simulink model "GMCLIB_ClarkInv_BAM_F32"  (Simulink 7.3)
settings: Solver=ode45  StartTime=0.0  StopTime=10.0  RelTol=1e-3
settings Model: Creator=B17364  LastModifiedBy=B17364

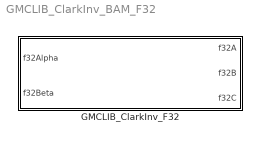
== system GMCLIB_ClarkInv_BAM_F32 ==
  GMCLIB_ClarkInv_F32 : Subsystem  mask(GMCLIB_ClarkInv_F32){}
      mask help: Bit accurate model of inverse Clarke transformation 2ph -> 3ph
      mask init:
      | pos = get_param(gcb, 'Position');width = pos(3) - pos(1); height = pos(4) - pos(2);tX=width/2;tY=height*0.9;
      mask Display: color('black');port_label('input',1,'f32Alpha');port_label('input',2,'f32Beta');port_label('output',1,'f32A');port_label('output',2,'f32B');port_label('output',3,'f32C');color('black');disp('GMCLIB_ClarkInv_F32');color('blue');text(tX,tY, 'BAM', 'horizontalAlignment', 'center');

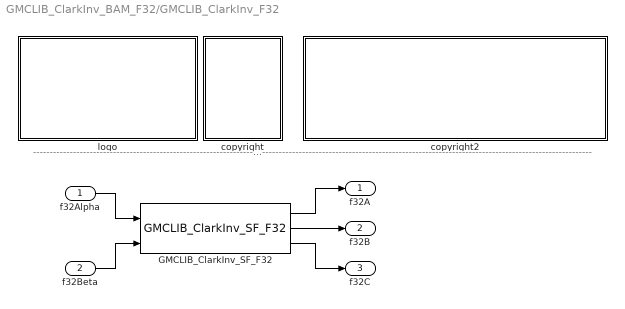
== system GMCLIB_ClarkInv_BAM_F32/GMCLIB_ClarkInv_F32 ==
  note: ---------------------------------------------------------------------------------------------------------------------------------------------------------------------------------------------------
  f32Alpha : Inport  OutDataType=fixdt(1, 16)  OutScaling=2^0
  f32Beta : Inport  Port=2  OutDataType=fixdt(1, 16)  OutScaling=2^0
  GMCLIB_ClarkInv_SF_F32 : S-Function  FunctionName=GMCLIB_ClarkInv_SF_F32  EnableBusSupport=off
  copyright : Subsystem
      mask Display: text(10,90,'FILE:');text(10,75,'DESRIPTION:')text(10,60,'COPYRIGHT:')text(10,45,'VERSION:')text(10,30,'DATE:')
  copyright2 : Subsystem
      mask Display: text(10,90,'GMCLIB_ClarkInv_BAM_F32.mdl');text(10,75,'Inverse Clarke transformation');text(10,60,'Freescale')text(10,45,'0.1');text(10,30,'30-Aug-2011');
  logo : Subsystem
      mask Display: image(imread('logo.jpg'))
  f32A : Outport  OutDataType=fixdt(1, 16)  OutScaling=2^0
  f32B : Outport  Port=2  OutDataType=fixdt(1, 16)  OutScaling=2^0
  f32C : Outport  Port=3  OutDataType=fixdt(1, 16)  OutScaling=2^0
  wires:
  f32Alpha/1 -> GMCLIB_ClarkInv_SF_F32/1
  f32Beta/1 -> GMCLIB_ClarkInv_SF_F32/2
  GMCLIB_ClarkInv_SF_F32/1 -> f32A/1
  GMCLIB_ClarkInv_SF_F32/2 -> f32B/1
  GMCLIB_ClarkInv_SF_F32/3 -> f32C/1

== system GMCLIB_ClarkInv_BAM_F32/GMCLIB_ClarkInv_F32/copyright ==

== system GMCLIB_ClarkInv_BAM_F32/GMCLIB_ClarkInv_F32/copyright2 ==

== system GMCLIB_ClarkInv_BAM_F32/GMCLIB_ClarkInv_F32/logo ==
